simulink model "LoadLevel1_VF"  (R2023a)
settings: Solver=ode23tb  StartTime=0.0  StopTime=250  MaxStep=0.02  RelTol=1e-3  AbsTol=1e-5
undefined symbols (not defined in the file): a, Ac, Bc, Cc, D1, Dc, Delta, find_system, Fnom, gcbh, I21_init_imag, I21_init_real, Ibase1, Ibase2, Iw1A_init_mag, Iw1A_init_pha, Iw1B_init_mag, Iw1B_init_pha, Iw1C_init_mag, Iw1C_init_pha, Iw2A_init_mag, Iw2A_init_pha, Iw2B_init_mag, Iw2B_init_pha, Iw2C_init_mag, Iw2C_init_pha, j, kr, ks, Nmax, Pnom, psi, RegulatorDeadBand, RegulatorDelay, RegulatorVref, sps_rtmsupport, Vnom1, Vnom2, w, Z1pu, Z2pu, Ztpu
libraries: spsThreePhaseVIMeasurementLib x15, spsThreePhasePISectionLineLib x14, spsThreePhaseParallelRLCLoadLib x11, spsControlledCurrentSourceLib x6, spsThreePhaseTransformerTwoWindingsLib x5, spsThreePhaseBreakerLib x2, spsExcitationSystemLib x2, spsHydraulicTurbineandGovernorLib x2, spsSynchronousMachinepuStandardLib x2, spsThreePhaseSeriesRLCBranchLib x2, spsGroundLib x2, spsSequenceAnalyzerPhasorLib x1
(part 2 of 3)

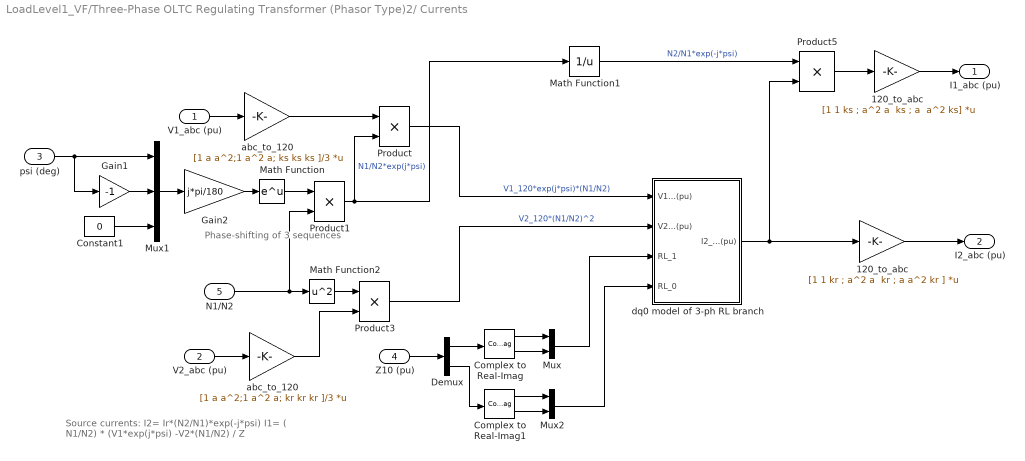
== system LoadLevel1_VF/Three-Phase OLTC Regulating Transformer (Phasor Type)2/ Currents  ==
  note: Phase-shifting
      | of 3 sequences
  note: Source currents:
      |
      | I2= Ir*(N2/N1)*exp(-j*psi)
      | I1= ( N1/N2) * (V1*exp(j*psi) -V2*(N1/N2) / Z
  V1_abc (pu) : Inport
  V2_abc (pu) : Inport  Port=2
  psi (deg) : Inport  Port=3
  Z10 (pu) : Inport  Port=4
  N1/N2 : Inport  Port=5
  120_to_abc : Gain  Gain="[1 1 kr ; a^2 a  kr ; a a^2 kr ]"  Multiplication=Matrix(K*u)  SaturateOnIntegerOverflow=on  OutDataTypeStr=Inherit: Same as input  ParamDataTypeStr=Inherit: Same as input
  "120_to_abc " : Gain  Gain="[1 1 ks ; a^2 a  ks ; a  a^2 ks]"  Multiplication=Matrix(K*u)  SaturateOnIntegerOverflow=on  OutDataTypeStr=Inherit: Same as input  ParamDataTypeStr=Inherit: Same as input
  Complex to Real-Imag : ComplexToRealImag
  Complex to Real-Imag1 : ComplexToRealImag
  Constant1 : Constant  Value=0
  Demux : Demux  Outputs=2
      settings: DisplayOption=none
  Gain1 : Gain  Gain=-1  SaturateOnIntegerOverflow=on  OutDataTypeStr=Inherit: Same as input  ParamDataTypeStr=Inherit: Same as input
  Gain2 : Gain  Gain=j*pi/180  SaturateOnIntegerOverflow=on  OutDataTypeStr=Inherit: Same as input  ParamDataTypeStr=Inherit: Same as input
  Math Function : Math  SignedPower=on
  Math Function1 : Math  Operator=reciprocal  SignedPower=on
  Math Function2 : Math  Operator=square  SignedPower=on
  Mux : Mux  Inputs=2
  Mux1 : Mux  Inputs=3
  Mux2 : Mux  Inputs=2
  Product : Product  SaturateOnIntegerOverflow=on  OutDataTypeStr=Inherit: Same as first input
  Product1 : Product  Inputs=**  SaturateOnIntegerOverflow=on  OutDataTypeStr=Inherit: Same as first input
  Product3 : Product  Inputs=**  SaturateOnIntegerOverflow=on  OutDataTypeStr=Inherit: Same as first input
  Product5 : Product  SaturateOnIntegerOverflow=on  OutDataTypeStr=Inherit: Same as first input
  abc_to_120 : Gain  Gain=[1 a a^2;1 a^2 a; ks ks ks ]/3  Multiplication=Matrix(K*u)  SaturateOnIntegerOverflow=on  OutDataTypeStr=Inherit: Same as input  ParamDataTypeStr=Inherit: Same as input
  "abc_to_120 " : Gain  Gain=[1 a a^2;1 a^2 a; kr kr kr ]/3  Multiplication=Matrix(K*u)  SaturateOnIntegerOverflow=on  OutDataTypeStr=Inherit: Same as input  ParamDataTypeStr=Inherit: Same as input
  dq0 model of 3-ph RL branch : Subsystem
  I1_abc (pu) : Outport  VectorParamsAs1DForOutWhenUnconnected=off
  "I2_abc (pu) " : Outport  Port=2  VectorParamsAs1DForOutWhenUnconnected=off
  wires:
  Gain2/1 -> Math Function/1
  Product/1 -> dq0 model of 3-ph RL branch/1(V1_120(pu))  "V1_120*exp(j*psi)*(N1/N2)"
  Product3/1 -> dq0 model of 3-ph RL branch/2(V2_120(pu))  "V2_120*(N1/N2)^2"
  N1/N2/1 -> Product1/2, Math Function2/1
  Product1/1 -> Math Function1/1, Product/2  "N1/N2*exp(j*psi)"
  Math Function/1 -> Product1/1
  V1_abc (pu)/1 -> abc_to_120/1
  V2_abc (pu)/1 -> "abc_to_120 "/1
  Product5/1 -> "120_to_abc "/1
  abc_to_120/1 -> Product/1
  Math Function1/1 -> Product5/1  "N2/N1*exp(-j*psi)"
  psi (deg)/1 -> Gain1/1, Mux1/1
  Mux1/1 -> Gain2/1
  Gain1/1 -> Mux1/2
  Constant1/1 -> Mux1/3
  "abc_to_120 "/1 -> Product3/2
  120_to_abc/1 -> "I2_abc (pu) "/1
  "120_to_abc "/1 -> I1_abc (pu)/1
  Z10 (pu)/1 -> Demux/1
  Demux/1 -> Complex to Real-Imag/1
  Demux/2 -> Complex to Real-Imag1/1
  Complex to Real-Imag/1 -> Mux/1
  Complex to Real-Imag/2 -> Mux/2
  Mux/1 -> dq0 model of 3-ph RL branch/3(RL_1)
  Complex to Real-Imag1/1 -> Mux2/1
  Complex to Real-Imag1/2 -> Mux2/2
  Mux2/1 -> dq0 model of 3-ph RL branch/4(RL_0)
  dq0 model of 3-ph RL branch/1(I2_120 (pu)) -> 120_to_abc/1, Product5/2
  Math Function2/1 -> Product3/1

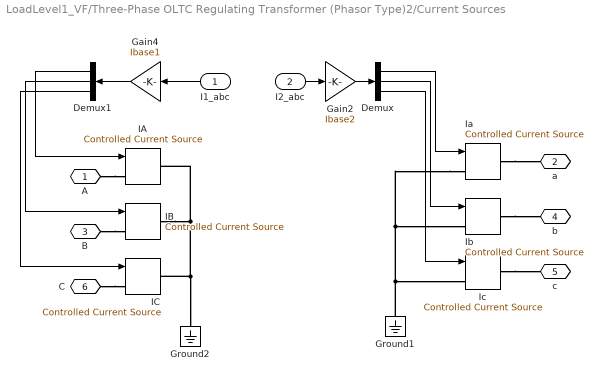
== system LoadLevel1_VF/Three-Phase OLTC Regulating Transformer (Phasor Type)2/Current Sources ==
  I1_abc : Inport
  I2_abc : Inport  Port=2
  Demux : Demux  Outputs=3
      settings: DisplayOption=none
  Demux1 : Demux  Outputs=3
      settings: DisplayOption=none
  Gain2 : Gain  Gain=Ibase2  SaturateOnIntegerOverflow=on  OutDataTypeStr=Inherit: Same as input  ParamDataTypeStr=Inherit: Same as input
  Gain4 : Gain  Gain=Ibase1  SaturateOnIntegerOverflow=on  OutDataTypeStr=Inherit: Same as input  ParamDataTypeStr=Inherit: Same as input
  Ground1 : spsGroundLib/Ground  LConnTagsString=a
  Ground2 : spsGroundLib/Ground  LConnTagsString=a
  IA : spsControlledCurrentSourceLib/Controlled Current Source  Initialize=on  Source_Type=AC  Amplitude=Iw1A_init_mag  Phase=Iw1A_init_pha  Frequency=Fnom  Measurements=None
  IB : spsControlledCurrentSourceLib/Controlled Current Source  Initialize=on  Source_Type=AC  Amplitude=Iw1B_init_mag  Phase=Iw1B_init_pha  Frequency=Fnom  Measurements=None
  IC : spsControlledCurrentSourceLib/Controlled Current Source  Initialize=on  Source_Type=AC  Amplitude=Iw1C_init_mag  Phase=Iw1C_init_pha  Frequency=Fnom  Measurements=None
  Ia : spsControlledCurrentSourceLib/Controlled Current Source  Initialize=on  Source_Type=AC  Amplitude=Iw2A_init_mag  Phase=Iw2A_init_pha  Frequency=Fnom  Measurements=None
  Ib : spsControlledCurrentSourceLib/Controlled Current Source  Initialize=on  Source_Type=AC  Amplitude=Iw2B_init_mag  Phase=Iw2B_init_pha  Frequency=Fnom  Measurements=None
  Ic : spsControlledCurrentSourceLib/Controlled Current Source  Initialize=on  Source_Type=AC  Amplitude=Iw2C_init_mag  Phase=Iw2C_init_pha  Frequency=Fnom  Measurements=None
  A : PMIOPort  Side=Left
  a : PMIOPort  Port=2  Side=Right
  B : PMIOPort  Port=3  Side=Left
  b : PMIOPort  Port=4  Side=Right
  c : PMIOPort  Port=5  Side=Right
  C : PMIOPort  Port=6  Side=Left
  wires:
  I1_abc/1 -> Gain4/1
  I2_abc/1 -> Gain2/1
  Demux/3 -> Ic/1
  Demux/2 -> Ib/1
  Demux/1 -> Ia/1
  Demux1/3 -> IC/1
  Demux1/2 -> IB/1
  Demux1/1 -> IA/1
  Gain2/1 -> Demux/1
  Gain4/1 -> Demux1/1
  connections:
  Ic/RConn1 -- c/RConn1
  Ib/RConn1 -- b/RConn1
  Ia/RConn1 -- a/RConn1
  C/RConn1 -- IC/LConn1
  B/RConn1 -- IB/LConn1
  A/RConn1 -- IA/LConn1
  Ia/LConn1 -- Ib/LConn1 -- Ic/LConn1 -- Ground1/LConn1
  IB/RConn1 -- IA/RConn1 -- IC/RConn1 -- Ground2/LConn1

== system LoadLevel1_VF/Three-Phase OLTC Regulating Transformer (Phasor Type)2/Tap Changer Control ==
  "Up " : Inport
  "Down " : Inport  Port=2
  Constant : Constant  Value=-1
  Constant1 : Constant
  Determine tap position : Subsystem
  Edge Detector : Subsystem  DialogController=POWERSYS.PowerSysDialog  mask(Edge Detector){model=Rising, ic=0}
      mask prompts: model "Edge:"; ic "Input at t = -eps:"
      mask help:
      | This block compares its present input to its previous input.
      |
      | If the input  is a logic signal (TRUE (1) or FALSE (0), the output is a one-step boolean signal TRUE  when  the specified edge (Rising, Falling or Either)  is detected.
      |
      | This block can also be used to detect the slope polarity of a continuous signal. For example, if the specified edge is  "Rising", the output is TRUE as long as the slope of the input signal is positive.
      |
      | The input value at time preceding t=0 is specified by the parameter "Input at t=-eps"
      mask init:
      | if model~=3,
      | 	x1 = (model -1)*20;
      |     x2 = (model -1)*60;
      | 	X1=[5,20,20,35]+25; Y1=[20+x2,20+x2,80-x2,80-x2];
      | 	X2=[5,20,35]+25;    Y2=[40+x1,60-x1,40+x1];
      | 	X3=[];X4=[];Y3=[];Y4=[];
      | else
      | 	x1 = 20;
      | 	x2 = 60;
      | 	X1=[5,20,20,35]+8; Y1=[20,20,80,80];
      | 	X2=[5,20,35]+8;    Y2=[40,60,40];
      | 	X3=[5,20,20,35]+53; Y3=[20+x2,20+x2,80-x2,80-x2];
      | 	X4=[5,20,35]+53;    Y4=[40+x1,60-x1,40+x1];
      | end
      | power_initmask();
      mask Help: This block is part of a subset of blocks in the Extras library that does not have documentation associated with it, other than the block mask description.
      mask TypeOptions model: Rising | Falling | Either
      mask Display: plot(0,0,100,100, X1,Y1,X2,Y2,X3,Y3,X4,Y4);
  Logical Operator : Logic  Operator=OR  AllPortsSameDT=off
  Logical Operator1 : Logic  AllPortsSameDT=off
  Mechanical Delay : TransportDelay  DelayTime=MecDelay  InitialOutput=InitialPosition
  Memory : Memory  InitialCondition=1  InheritSampleTime=on
  Relational Operator : RelationalOperator  Operator===  OutDataTypeStr=float('double')  InputSameDT=off
  Switch : Switch  Threshold=0.5  InputSameDT=off
  TapNo : Outport  VectorParamsAs1DForOutWhenUnconnected=off
  Ready : Outport  Port=2  VectorParamsAs1DForOutWhenUnconnected=off
  wires:
  Edge Detector/1(Out) -> Logical Operator1/2
  Logical Operator/1 -> Edge Detector/1(In)
  Memory/1 -> Ready/1, Logical Operator1/1
  Relational Operator/1 -> Memory/1
  Determine tap position/1(TapNo) -> Relational Operator/1, Mechanical Delay/1
  Switch/1 -> Determine tap position/1(NewTap)
  Constant1/1 -> Switch/3
  Constant/1 -> Switch/1
  "Down "/1 -> Switch/2, Logical Operator/2
  "Up "/1 -> Logical Operator/1
  Logical Operator1/1 -> Determine tap position/Trigger
  Mechanical Delay/1 -> Relational Operator/2, TapNo/1

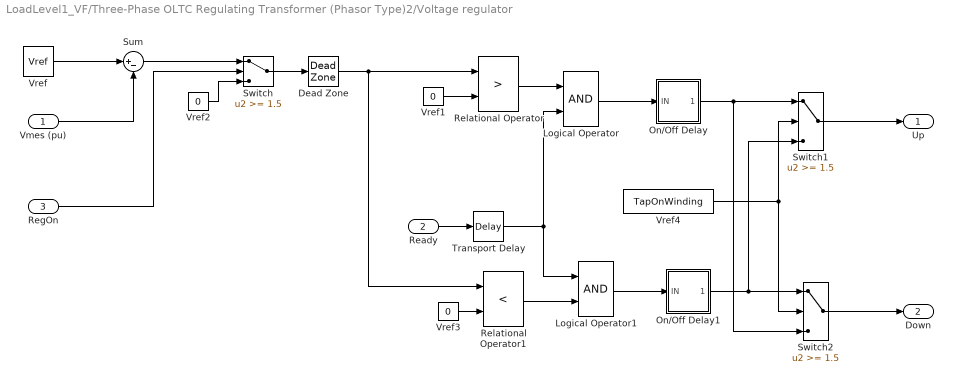
== system LoadLevel1_VF/Three-Phase OLTC Regulating Transformer (Phasor Type)2/Voltage regulator ==
  Vmes (pu) : Inport
  Ready : Inport  Port=2
  RegOn : Inport  Port=3
  Dead Zone : DeadZone  LowerValue=-DeadBand/2  UpperValue=+DeadBand/2
  Logical Operator : Logic  AllPortsSameDT=off
  Logical Operator1 : Logic  AllPortsSameDT=off
  On/Off Delay : Subsystem  DialogController=POWERSYS.PowerSysDialog  mask(On/Off Delay){type_delay=On delay, delay=TimeDelay, ic=0}
      mask prompts: type_delay "Type:"; delay "Time delay:"; ic "Input at t = -eps (0/1):"
      mask help:
      | Apply a delay on the input signal when the input changes to TRUE (1) or FALSE (0).
      |
      | On delay: When the input becomes TRUE, the output becomes TRUE after the specified time delay as long as the input is still TRUE. If the input becomes FALSE before the time delay has expired , the output stays FALSE.
      |
      | Off delay: When the input becomes FALSE, the output becomes FALSE after the specified time delay as long as the input is still FALSE. If the input becomes TRUE before the time delay has expired , the output stays TRUE.
      |
      | The input value (0/1) at time preceding t=0 is specified by the parameter "input at t = -eps".
      mask init:
      | str=sprintf('%g %c',delay,'s');
      | power_initmask();
      mask Help: This block is part of a subset of blocks in the Extras library that does not have documentation associated with it, other than the block mask description.
      mask TypeOptions type_delay: On delay | Off delay
      mask Display:
      | plot(0,0,100,100,[10,10,10,90,90,90],[60,40,50,50,40,60]);
      | text(25+(type_delay-1)*50,80,'t');
      | text(15,20,str);
  On/Off Delay1 : Subsystem  DialogController=POWERSYS.PowerSysDialog  mask(On/Off Delay){type_delay=On delay, delay=TimeDelay, ic=0}
      mask prompts: type_delay "Type:"; delay "Time delay:"; ic "Input at t = -eps (0/1):"
      mask help:
      | Apply a delay on the input signal when the input changes to TRUE (1) or FALSE (0).
      |
      | On delay: When the input becomes TRUE, the output becomes TRUE after the specified time delay as long as the input is still TRUE. If the input becomes FALSE before the time delay has expired , the output stays FALSE.
      |
      | Off delay: When the input becomes FALSE, the output becomes FALSE after the specified time delay as long as the input is still FALSE. If the input becomes TRUE before the time delay has expired , the output stays TRUE.
      |
      | The input value (0/1) at time preceding t=0 is specified by the parameter "input at t = -eps".
      mask init:
      | str=sprintf('%g %c',delay,'s');
      | power_initmask();
      mask Help: This block is part of a subset of blocks in the Extras library that does not have documentation associated with it, other than the block mask description.
      mask TypeOptions type_delay: On delay | Off delay
      mask Display:
      | plot(0,0,100,100,[10,10,10,90,90,90],[60,40,50,50,40,60]);
      | text(25+(type_delay-1)*50,80,'t');
      | text(15,20,str);
  Relational Operator : RelationalOperator  Operator=>  InputSameDT=off
  Relational Operator1 : RelationalOperator  Operator=<  InputSameDT=off
  Sum : Sum  Inputs=|+-  SaturateOnIntegerOverflow=on
  Switch : Switch  Threshold=1.5  InputSameDT=off
  Switch1 : Switch  Threshold=1.5  InputSameDT=off
  Switch2 : Switch  Threshold=1.5  InputSameDT=off
  Transport Delay : TransportDelay  DelayTime=3/60  InitialOutput=1
  Vref : Constant  Value=Vref
  Vref1 : Constant  Value=0
  Vref2 : Constant  Value=0
  Vref3 : Constant  Value=0
  Vref4 : Constant  Value=TapOnWinding
  "Up " : Outport  VectorParamsAs1DForOutWhenUnconnected=off
  "Down " : Outport  Port=2  VectorParamsAs1DForOutWhenUnconnected=off
  wires:
  Vref4/1 -> Switch2/2, Switch1/2
  Switch2/1 -> "Down "/1
  On/Off Delay1/1(OUT) -> Switch1/3, Switch2/1
  Switch1/1 -> "Up "/1
  On/Off Delay/1(OUT) -> Switch2/3, Switch1/1
  Vref2/1 -> Switch/3
  RegOn/1 -> Switch/2
  Switch/1 -> Dead Zone/1
  Sum/1 -> Switch/1
  Vref/1 -> Sum/1
  Vmes (pu)/1 -> Sum/2
  Dead Zone/1 -> Relational Operator1/1, Relational Operator/1
  Vref1/1 -> Relational Operator/2
  Relational Operator/1 -> Logical Operator/1
  Ready/1 -> Transport Delay/1
  Logical Operator/1 -> On/Off Delay/1(IN)
  Transport Delay/1 -> Logical Operator/2, Logical Operator1/1
  Vref3/1 -> Relational Operator1/2
  Relational Operator1/1 -> Logical Operator1/2
  Logical Operator1/1 -> On/Off Delay1/1(IN)

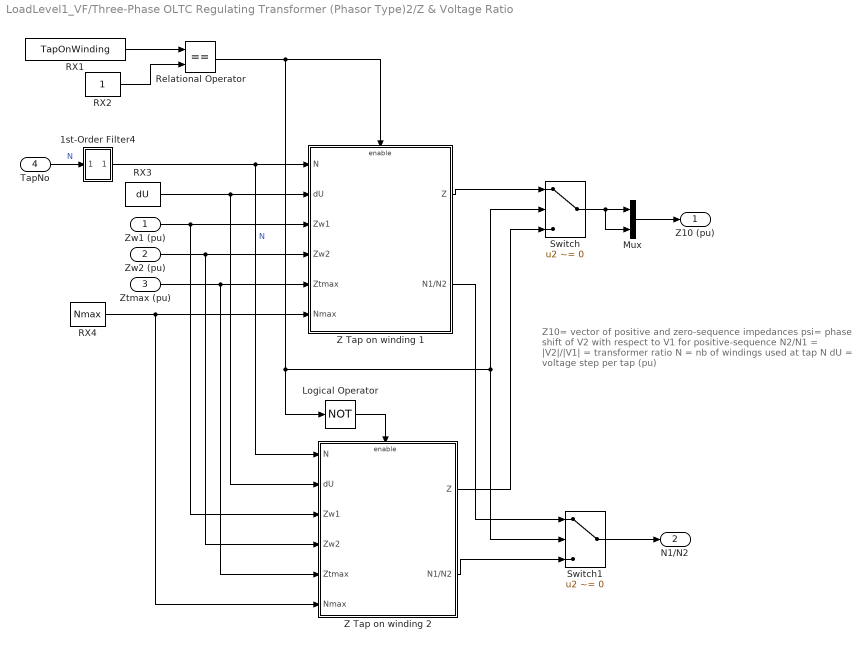
== system LoadLevel1_VF/Three-Phase OLTC Regulating Transformer (Phasor Type)2/Z & Voltage Ratio ==
  note: Z10= vector of positive and zero-sequence impedances
      | psi= phase shift of  V2 with respect to V1 for positive-sequence
      | N2/N1 =  |V2|/|V1| = transformer ratio
      | N = nb of windings used at tap N
      | dU = voltage step  per tap (pu)
  Zw1 (pu) : Inport
  Zw2 (pu) : Inport  Port=2
  Ztmax (pu) : Inport  Port=3
  TapNo : Inport  Port=4
  1st-Order Filter4 : Subsystem  DialogController=POWERSYS.PowerSysDialog  mask(First-Order Filter){FilterType=Lowpass, Tc=1/Fnom, Initialize=on, Vac_Init=[0 0  Fnom], Vdc_Init=InitialTap, PlotResponse=off, param1=[1 500 1]}
      mask prompts: FilterType "Filter Type:"; Tc "Time constant (s):"; Initialize "Initialize filter states"; Vac_Init "AC initial input: [ Mag  Phase(degrees)  Freq(Hz) ]"; Vdc_Init "DC Initial input:"; PlotResponse "Plot filter response"; param1 "Frequency range(Hz) : [Start  End  Inc.]"
      mask init:
      | switch FilterType
      | case 1, % Lowpass
      |        X=[0 1 2 3 4];
      |        Y=[-2 -2 -3 -4 -4];
      |        numc=1;
      |        denc=[Tc 1];
      |  case 2,   % Highpass
      |        X=[0 1 2 3 4];
      |        Y=[-4 -4 -3 -2 -2];
      |         numc=[1 0];
      |         denc=[1 1/Tc];
      | end
      | %
      | [Ac,Bc,Cc,Dc]=tf2ss(numc,denc);
      | %
      | %
      | if Initialize==1  % Compute initial conditions on states
      | u1=Vac_Init(1)*exp(j*Vac_Init(2)*pi/180);
      | u2=Vdc_Init*exp(j*90*pi/180);
      | u=u1+u2;
      | u0=imag(u); % input at  t=0;
      | I=eye(size(Ac));
      | sI1=I*j*(2*pi*Vac_Init(3));
      | sI2=I*j*0;
      | x=inv(sI1-Ac)*Bc*u1 + inv(sI2-Ac)*Bc*u2;
      | x0c=imag(x);
      | else
      | x0c=0;
      | end
      | %
      | if PlotResponse==1 % Plot frequency and step response
      | t=[0:Tc/1000:7*Tc];
      | f=param1(1):param1(3):param1(2);
      | w=2*pi*f;
      | switch FilterType
      | 	case 1, % Lowpass
      | 		Ystep=1 - exp(-t/Tc);
      | 		RepFreq=1./(1+Tc*j.*w);
      | 	case 2,   % Highpass
      | 		Ystep=exp(-t/Tc);
      | 		RepFreq=1./(1 + (1./(Tc*j.*w)));
      | end
      | %
      | Mag=abs(RepFreq);
      | Pha=angle(RepFreq)*180/pi;
      | %
      | figure(1)
      | subplot(2,1,1)
      | plot(f,Mag)
      | grid
      | title('Bode Diagram')
      | ylabel('Magnitude')
      | subplot(2,1,2)
      | plot(f,Pha)
      | ylabel('Phase (deg)')
      | xlabel('Frequency (Hz)')
      | grid
      | figure(2)
      | plot(t,Ystep)
      | grid
      | ylabel('Amplitude')
      | xlabel('Time (s)')
      | title('Step Response')
      | end
      | power_initmask();
      mask Help: This block is part of a subset of blocks in the Extras library that does not have documentation associated with it, other than the block mask description.
      mask TypeOptions FilterType: Lowpass | Highpass
      mask Callback Initialize: %parametres=get_param(gcb,'MaskValues');p3=parametres{3};p6=parametres{6};if strcmp(p3,'on');param4='on';param5='on';else;param4='off';param5='off';end;if strcmp(p6,'on');param7='on';else;param7='off';end;visible={'on','on','on',param4,param5,'on',param7};set_param(gcb,'MaskVisibilities',visible)
      mask Callback PlotResponse: %parametres=get_param(gcb,'MaskValues');p3=parametres{3};p6=parametres{6};if strcmp(p3,'on');param4='on';param5='on';else;param4='off';param5='off';end;if strcmp(p6,'on');param7='on';else;param7='off';end;visible={'on','on','on',param4,param5,'on',param7};set_param(gcb,'MaskVisibilities',visible)
      mask Display: plot(X,Y);
  Logical Operator : Logic  Operator=NOT  AllPortsSameDT=off
  Mux : Mux  Inputs=2
  RX1 : Constant  Value=TapOnWinding
  RX2 : Constant
  RX3 : Constant  Value=dU
  RX4 : Constant  Value=Nmax
  Relational Operator : RelationalOperator  Operator===  InputSameDT=off
  Switch : Switch  Criteria=u2 ~= 0  Threshold=0.5  InputSameDT=off
  Switch1 : Switch  Criteria=u2 ~= 0  Threshold=0.5  InputSameDT=off
  Z Tap on winding 1 : Subsystem
  Z Tap on winding 2 : Subsystem
  "Z10 (pu) " : Outport  VectorParamsAs1DForOutWhenUnconnected=off
  N1/N2 : Outport  Port=2  VectorParamsAs1DForOutWhenUnconnected=off
  wires:
  RX4/1 -> Z Tap on winding 2/6(Nmax), Z Tap on winding 1/6(Nmax)
  TapNo/1 -> 1st-Order Filter4/1(In)  "N"
  1st-Order Filter4/1(Out) -> Z Tap on winding 1/1(N), Z Tap on winding 2/1(N)  "N"
  Zw2 (pu)/1 -> Z Tap on winding 1/4(Zw2), Z Tap on winding 2/4(Zw2)
  Zw1 (pu)/1 -> Z Tap on winding 1/3(Zw1), Z Tap on winding 2/3(Zw1)
  RX1/1 -> Relational Operator/1
  RX2/1 -> Relational Operator/2
  Relational Operator/1 -> Z Tap on winding 1/Enable, Logical Operator/1, Switch/2, Switch1/2
  Logical Operator/1 -> Z Tap on winding 2/Enable
  Z Tap on winding 1/1(Z) -> Switch/1
  Z Tap on winding 2/1(Z) -> Switch/3
  Z Tap on winding 1/2(N1/N2) -> Switch1/1
  Z Tap on winding 2/2(N1/N2) -> Switch1/3
  Switch1/1 -> N1/N2/1
  Ztmax (pu)/1 -> Z Tap on winding 1/5(Ztmax), Z Tap on winding 2/5(Ztmax)
  RX3/1 -> Z Tap on winding 1/2(dU), Z Tap on winding 2/2(dU)
  Switch/1 -> Mux/1, Mux/2
  Mux/1 -> "Z10 (pu) "/1

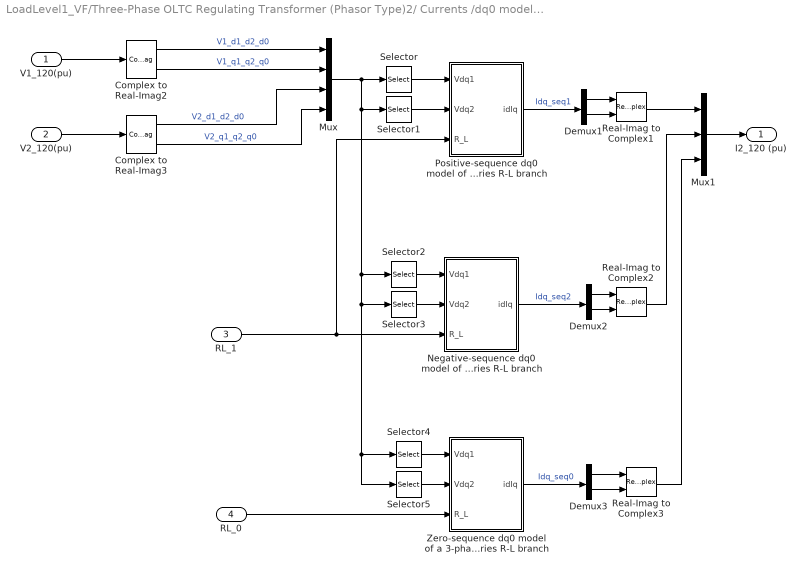
== system LoadLevel1_VF/Three-Phase OLTC Regulating Transformer (Phasor Type)2/ Currents /dq0 model of 3-ph RL branch ==
  V1_120(pu) : Inport
  V2_120(pu) : Inport  Port=2
  RL_1 : Inport  Port=3
  RL_0 : Inport  Port=4
  Complex to Real-Imag2 : ComplexToRealImag
  Complex to Real-Imag3 : ComplexToRealImag
  Demux1 : Demux  Outputs=2
      settings: DisplayOption=none
  Demux2 : Demux  Outputs=2
      settings: DisplayOption=none
  Demux3 : Demux  Outputs=2
      settings: DisplayOption=none
  Mux : Mux
  Mux1 : Mux  Inputs=3
  Negative-sequence dq0 model of a 3-phase series R-L branch : Subsystem
  Positive-sequence dq0 model of a 3-phase series R-L branch : Subsystem
  Real-Imag to Complex1 : RealImagToComplex
  Real-Imag to Complex2 : RealImagToComplex
  Real-Imag to Complex3 : RealImagToComplex
  Selector : Selector  InputPortWidth=12  IndexOptions=Index vector (dialog)  Indices=[1 4]  OutputSizes=1
  Selector1 : Selector  InputPortWidth=12  IndexOptions=Index vector (dialog)  Indices=[7 10]  OutputSizes=1
  Selector2 : Selector  InputPortWidth=12  IndexOptions=Index vector (dialog)  Indices=[1 4]+1  OutputSizes=1
  Selector3 : Selector  InputPortWidth=12  IndexOptions=Index vector (dialog)  Indices=[7 10]+1  OutputSizes=1
  Selector4 : Selector  InputPortWidth=12  IndexOptions=Index vector (dialog)  Indices=[1 4]+2  OutputSizes=1
  Selector5 : Selector  InputPortWidth=12  IndexOptions=Index vector (dialog)  Indices=[7 10]+2  OutputSizes=1
  Zero-sequence dq0 model of a 3-phase series R-L branch : Subsystem
  I2_120 (pu) : Outport  VectorParamsAs1DForOutWhenUnconnected=off
  wires:
  Positive-sequence dq0 model of a 3-phase series R-L branch/1(idIq) -> Demux1/1  "Idq_seq1"
  V1_120(pu)/1 -> Complex to Real-Imag2/1
  V2_120(pu)/1 -> Complex to Real-Imag3/1
  Selector/1 -> Positive-sequence dq0 model of a 3-phase series R-L branch/1(Vdq1)
  Selector1/1 -> Positive-sequence dq0 model of a 3-phase series R-L branch/2(Vdq2)
  Mux/1 -> Selector/1, Selector1/1, Selector2/1, Selector3/1, Selector4/1, Selector5/1
  Selector2/1 -> Negative-sequence dq0 model of a 3-phase series R-L branch/1(Vdq1)
  Selector3/1 -> Negative-sequence dq0 model of a 3-phase series R-L branch/2(Vdq2)
  Selector4/1 -> Zero-sequence dq0 model of a 3-phase series R-L branch/1(Vdq1)
  Negative-sequence dq0 model of a 3-phase series R-L branch/1(idIq) -> Demux2/1  "Idq_seq2"
  Zero-sequence dq0 model of a 3-phase series R-L branch/1(idIq) -> Demux3/1  "Idq_seq0"
  Complex to Real-Imag2/1 -> Mux/1  "V1_d1_d2_d0"
  Complex to Real-Imag2/2 -> Mux/2  "V1_q1_q2_q0"
  Complex to Real-Imag3/1 -> Mux/3  "V2_d1_d2_d0"
  Complex to Real-Imag3/2 -> Mux/4  "V2_q1_q2_q0"
  RL_1/1 -> Positive-sequence dq0 model of a 3-phase series R-L branch/3(R_L), Negative-sequence dq0 model of a 3-phase series R-L branch/3(R_L)
  Selector5/1 -> Zero-sequence dq0 model of a 3-phase series R-L branch/2(Vdq2)
  RL_0/1 -> Zero-sequence dq0 model of a 3-phase series R-L branch/3(R_L)
  Demux1/2 -> Real-Imag to Complex1/2
  Demux1/1 -> Real-Imag to Complex1/1
  Real-Imag to Complex1/1 -> Mux1/1
  Demux2/2 -> Real-Imag to Complex2/2
  Demux2/1 -> Real-Imag to Complex2/1
  Real-Imag to Complex2/1 -> Mux1/2
  Demux3/2 -> Real-Imag to Complex3/2
  Demux3/1 -> Real-Imag to Complex3/1
  Real-Imag to Complex3/1 -> Mux1/3
  Mux1/1 -> I2_120 (pu)/1

== system LoadLevel1_VF/Three-Phase OLTC Regulating Transformer (Phasor Type)2/Tap Changer Control/Determine tap position ==
  NewTap : Inport
  Trigger : TriggerPort  VariantControl=Variant
  Memory : Memory  InitialCondition=InitialPosition  InheritSampleTime=on
  Saturation : Saturate  UpperLimit=MinMaxTap(2)  LowerLimit=MinMaxTap(1)
  Sum : Sum  Inputs=|++  SaturateOnIntegerOverflow=on
  TapNo : Outport  InitialOutput=InitialPosition  VectorParamsAs1DForOutWhenUnconnected=off
  wires:
  Saturation/1 -> Memory/1, TapNo/1
  Memory/1 -> Sum/2
  Sum/1 -> Saturation/1
  NewTap/1 -> Sum/1

== system LoadLevel1_VF/Three-Phase OLTC Regulating Transformer (Phasor Type)2/Tap Changer Control/Edge Detector ==
  note: Edge or Slope Detector
  In : Inport
  Constant1 : Constant  Value=model
  Demux : Demux  Outputs=2
      settings: DisplayOption=none
  Logical Operator1 : Logic  Operator=OR
  Memory : Memory  InitialCondition=ic  LinearizeAsDelay=on
  Multiport Switch : MultiPortSwitch  InputSameDT=off
  NEGATIVE Edge : Subsystem  TreatAsAtomicUnit=on
  POSITIVE Edge : Subsystem  TreatAsAtomicUnit=on
  either edge : Constant  Value=[1 1]
  neg. edge : Constant  Value=[0 1]
  pos. edge : Constant  Value=[1 0]
  Out : Outport  VectorParamsAs1DForOutWhenUnconnected=off
  wires:
  Logical Operator1/1 -> Out/1
  NEGATIVE Edge/1(OUT) -> Logical Operator1/2
  POSITIVE Edge/1(OUT) -> Logical Operator1/1
  Memory/1 -> POSITIVE Edge/2(IN previous), NEGATIVE Edge/2(IN previous)
  In/1 -> POSITIVE Edge/1(IN), NEGATIVE Edge/1(IN), Memory/1
  pos. edge/1 -> Multiport Switch/2
  neg. edge/1 -> Multiport Switch/3
  Constant1/1 -> Multiport Switch/1
  Multiport Switch/1 -> Demux/1
  Demux/1 -> POSITIVE Edge/Enable
  Demux/2 -> NEGATIVE Edge/Enable
  either edge/1 -> Multiport Switch/4

== system LoadLevel1_VF/Three-Phase OLTC Regulating Transformer (Phasor Type)2/Voltage regulator/On//Off Delay ==
  note: Silvano Casoria
      | Power System Simulation Laboratory
      | IREQ, Hydro-Quebc
  note: On/Off Delay
  IN : Inport
  Clock : Clock
  Constant : Constant
  Constant1 : Constant  Value=delay
  Constant2 : Constant  Value=type_delay
  Data Type Conversion1 : DataTypeConversion  OutDataTypeStr=boolean
  Logical Operator1 : Logic  Operator=OR
  Logical Operator2 : Logic  Operator=NOT  Inputs=1
  OFF Delay : Subsystem  TreatAsAtomicUnit=on
  ON Delay : Subsystem  TreatAsAtomicUnit=on
  Relational Operator1 : RelationalOperator  Operator===
  OUT : Outport  VectorParamsAs1DForOutWhenUnconnected=off
  wires:
  Data Type Conversion1/1 -> OFF Delay/1(IN), ON Delay/1(IN)
  Constant/1 -> Relational Operator1/2
  Relational Operator1/1 -> ON Delay/Enable, Logical Operator2/1
  Constant2/1 -> Relational Operator1/1
  Logical Operator2/1 -> OFF Delay/Enable
  OFF Delay/1(OUT) -> Logical Operator1/2
  ON Delay/1(OUT) -> Logical Operator1/1
  Logical Operator1/1 -> OUT/1
  Constant1/1 -> ON Delay/3(DELAY), OFF Delay/3(DELAY)
  IN/1 -> Data Type Conversion1/1
  Clock/1 -> OFF Delay/2(clock), ON Delay/2(clock)

== system LoadLevel1_VF/Three-Phase OLTC Regulating Transformer (Phasor Type)2/Voltage regulator/On//Off Delay1 ==
  note: Silvano Casoria
      | Power System Simulation Laboratory
      | IREQ, Hydro-Quebc
  note: On/Off Delay
  IN : Inport
  Clock : Clock
  Constant : Constant
  Constant1 : Constant  Value=delay
  Constant2 : Constant  Value=type_delay
  Data Type Conversion1 : DataTypeConversion  OutDataTypeStr=boolean
  Logical Operator1 : Logic  Operator=OR
  Logical Operator2 : Logic  Operator=NOT  Inputs=1
  OFF Delay : Subsystem  TreatAsAtomicUnit=on
  ON Delay : Subsystem  TreatAsAtomicUnit=on
  Relational Operator1 : RelationalOperator  Operator===
  OUT : Outport  VectorParamsAs1DForOutWhenUnconnected=off
  wires:
  Data Type Conversion1/1 -> OFF Delay/1(IN), ON Delay/1(IN)
  Constant/1 -> Relational Operator1/2
  Relational Operator1/1 -> ON Delay/Enable, Logical Operator2/1
  Constant2/1 -> Relational Operator1/1
  Logical Operator2/1 -> OFF Delay/Enable
  OFF Delay/1(OUT) -> Logical Operator1/2
  ON Delay/1(OUT) -> Logical Operator1/1
  Logical Operator1/1 -> OUT/1
  Constant1/1 -> ON Delay/3(DELAY), OFF Delay/3(DELAY)
  IN/1 -> Data Type Conversion1/1
  Clock/1 -> OFF Delay/2(clock), ON Delay/2(clock)

== system LoadLevel1_VF/Three-Phase OLTC Regulating Transformer (Phasor Type)2/Z & Voltage Ratio/1st-Order Filter4 ==
  In : Inport
  State-Space : StateSpace  A=Ac  B=Bc  C=Cc  D=Dc  InitialCondition=x0c
  Out : Outport  InitialOutput=0  VectorParamsAs1DForOutWhenUnconnected=off
  wires:
  In/1 -> State-Space/1
  State-Space/1 -> Out/1

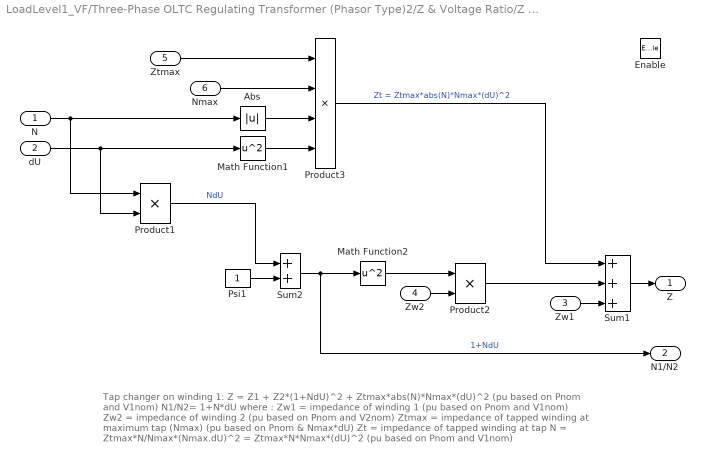
== system LoadLevel1_VF/Three-Phase OLTC Regulating Transformer (Phasor Type)2/Z & Voltage Ratio/Z Tap on winding 1 ==
  note: Tap changer on winding 1:
      | Z = Z1  + Z2*(1+NdU)^2 +  Ztmax*abs(N)*Nmax*(dU)^2       (pu based on Pnom and V1nom)
      | N1/N2= 1+N*dU
      |
      | where :
      | Zw1   =  impedance of winding 1 (pu based on Pnom and V1nom)
      | Zw2   =  impedance of winding 2 (pu based on Pnom and V2nom)
      | Ztmax =   impedance of tapped winding at maximum tap (Nmax)     (pu  based on  Pnom & Nmax*dU)
      | Zt =  impedance of tapped winding at tap N
      |      = Ztmax*N/Nmax*(Nmax.dU)^2 = Ztmax*N*Nmax*(dU)^2              (pu based on Pnom and V1nom)
  N : Inport
  dU : Inport  Port=2
  Zw1 : Inport  Port=3
  Zw2 : Inport  Port=4
  Ztmax : Inport  Port=5
  Nmax : Inport  Port=6
  Enable : EnablePort  PropagateVarSize=During execution
  Abs : Abs  SaturateOnIntegerOverflow=off
  Math Function1 : Math  Operator=square  SignedPower=on
  Math Function2 : Math  Operator=square  SignedPower=on
  Product1 : Product  SaturateOnIntegerOverflow=on  OutDataTypeStr=Inherit: Same as first input
  Product2 : Product  SaturateOnIntegerOverflow=on  OutDataTypeStr=Inherit: Same as first input
  Product3 : Product  Inputs=****  SaturateOnIntegerOverflow=on  OutDataTypeStr=Inherit: Same as first input
  Psi1 : Constant
  Sum1 : Sum  Inputs=+++  SaturateOnIntegerOverflow=on
  Sum2 : Sum  SaturateOnIntegerOverflow=on
  Z : Outport  VectorParamsAs1DForOutWhenUnconnected=off
  N1/N2 : Outport  Port=2  VectorParamsAs1DForOutWhenUnconnected=off
  wires:
  Nmax/1 -> Product3/2
  Math Function1/1 -> Product3/4
  Ztmax/1 -> Product3/1
  Product2/1 -> Sum1/2
  Math Function2/1 -> Product2/1
  Sum1/1 -> Z/1
  Zw2/1 -> Product2/2
  Zw1/1 -> Sum1/3
  Psi1/1 -> Sum2/2
  Sum2/1 -> Math Function2/1, N1/N2/1  "1+NdU"
  N/1 -> Product1/1, Abs/1
  dU/1 -> Product1/2, Math Function1/1
  Product1/1 -> Sum2/1  "NdU"
  Product3/1 -> Sum1/1  "Zt = Ztmax*abs(N)*Nmax*(dU)^2"
  Abs/1 -> Product3/3

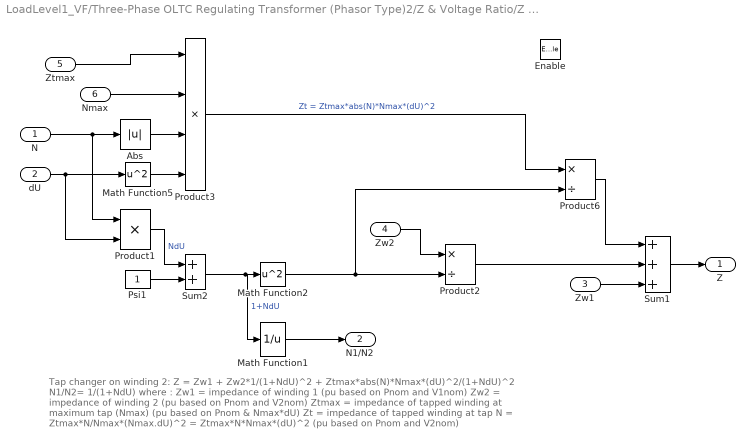
== system LoadLevel1_VF/Three-Phase OLTC Regulating Transformer (Phasor Type)2/Z & Voltage Ratio/Z Tap on winding 2 ==
  note: Tap changer on winding 2:
      | Z = Zw1  + Zw2*1/(1+NdU)^2 +  Ztmax*abs(N)*Nmax*(dU)^2/(1+NdU)^2
      | N1/N2= 1/(1+NdU)
      |
      | where :
      | Zw1   =  impedance of winding 1 (pu based on Pnom and V1nom)
      | Zw2   =  impedance of winding 2 (pu based on Pnom and V2nom)
      | Ztmax = impedance of tapped winding at maximum tap (Nmax)     (pu  based on  Pnom & Nmax*dU)
      | Zt =  impedance of tapped winding at tap N
      |      = Ztmax*N/Nmax*(Nmax.dU)^2 = Ztmax*N*Nmax*(dU)^2             (pu based on Pnom and V2nom)
  N : Inport
  dU : Inport  Port=2
  Zw1 : Inport  Port=3
  Zw2 : Inport  Port=4
  Ztmax : Inport  Port=5
  Nmax : Inport  Port=6
  Enable : EnablePort  PropagateVarSize=During execution
  Abs : Abs  SaturateOnIntegerOverflow=off
  Math Function1 : Math  Operator=reciprocal  SignedPower=on
  Math Function2 : Math  Operator=square  SignedPower=on
  Math Function5 : Math  Operator=square  SignedPower=on
  Product1 : Product  SaturateOnIntegerOverflow=on  OutDataTypeStr=Inherit: Same as first input
  Product2 : Product  Inputs=*/  SaturateOnIntegerOverflow=on  OutDataTypeStr=Inherit: Same as first input
  Product3 : Product  Inputs=****  SaturateOnIntegerOverflow=on  OutDataTypeStr=Inherit: Same as first input
  Product6 : Product  Inputs=*/  SaturateOnIntegerOverflow=on  OutDataTypeStr=Inherit: Same as first input
  Psi1 : Constant
  Sum1 : Sum  Inputs=+++  SaturateOnIntegerOverflow=on
  Sum2 : Sum  SaturateOnIntegerOverflow=on
  Z : Outport  VectorParamsAs1DForOutWhenUnconnected=off
  N1/N2 : Outport  Port=2  VectorParamsAs1DForOutWhenUnconnected=off
  wires:
  Math Function5/1 -> Product3/4
  Nmax/1 -> Product3/2
  Ztmax/1 -> Product3/1
  Product1/1 -> Sum2/1  "NdU"
  dU/1 -> Product1/2, Math Function5/1
  N/1 -> Product1/1, Abs/1
  Sum2/1 -> Math Function2/1, Math Function1/1  "1+NdU"
  Psi1/1 -> Sum2/2
  Zw1/1 -> Sum1/3
  Sum1/1 -> Z/1
  Product2/1 -> Sum1/2
  Zw2/1 -> Product2/1
  Math Function2/1 -> Product2/2, Product6/2
  Product3/1 -> Product6/1  "Zt = Ztmax*abs(N)*Nmax*(dU)^2"
  Product6/1 -> Sum1/1
  Math Function1/1 -> N1/N2/1
  Abs/1 -> Product3/3

== system LoadLevel1_VF/Three-Phase OLTC Regulating Transformer (Phasor Type)2/ Currents /dq0 model of 3-ph RL branch/Negative-sequence dq0 model of a 3-phase series R-L branch ==
  note: where w = 2*pi*Fnom (Hz)
  note: Vq1 - Vq2 = [ R * Iq ] + [ L* w * Id ] + [ L * d/dt (Iq) ]
  note: ==========================================================================================
  note: I --->
  note: V2
  note: V1
  note: o--------| R |---| L |-------o
  note: Vd1 - Vd2 = [ R * Id ] - [ L* w * Iq ] + [ L * d/dt (Id) ]
  note: where w = 2*pi*Fnom (Hz)
  note: Iq = [ w / ( L * s ) ] * [ Vq1 - Vq2 - ( R * Iq ) - ( L * Id ) ]
  note: Id = [ w / ( L * s ) ] * [ Vd1 - Vd2 - ( R * Id ) + ( L * Iq ) ]
  note: d-q axis model of a 3-phase series R-L branch
  note: Using Laplace transform and per unit (pu) quantities :
  Vdq1 : Inport
  Vdq2 : Inport  Port=2
  R_L : Inport  Port=3
  Demux3 : Demux  Outputs=2
      settings: DisplayOption=none
  Integrator : Integrator
  Product : Product  SaturateOnIntegerOverflow=on  OutDataTypeStr=Inherit: Same as first input
  Product1 : Product  SaturateOnIntegerOverflow=on  OutDataTypeStr=Inherit: Same as first input
  Product2 : Product  Inputs=*/  SaturateOnIntegerOverflow=on  OutDataTypeStr=Inherit: Same as first input
  R_choke2 : Gain  Gain=[1 -1]  SaturateOnIntegerOverflow=on  OutDataTypeStr=Inherit: Same as input  ParamDataTypeStr=Inherit: Same as input
  R_choke3 : Gain  Gain=w  SaturateOnIntegerOverflow=on  OutDataTypeStr=Inherit: Same as input  ParamDataTypeStr=Inherit: Same as input
  Selector : Selector  InputPortWidth=2  IndexOptions=Index vector (dialog)  Indices=[2 1]  OutputSizes=1
  Sum : Sum  Inputs=+--+  SaturateOnIntegerOverflow=on
  idIq : Outport  VectorParamsAs1DForOutWhenUnconnected=off
  wires:
  Demux3/1 -> Product/2
  Demux3/2 -> Product1/2, Product2/2
  R_L/1 -> Demux3/1
  Product2/1 -> Integrator/1
  R_choke3/1 -> Product2/1
  Selector/1 -> Product1/1
  Integrator/1 -> Product/1, Selector/1, idIq/1
  Sum/1 -> R_choke3/1
  Product1/1 -> R_choke2/1
  R_choke2/1 -> Sum/4
  Product/1 -> Sum/3
  Vdq2/1 -> Sum/2
  Vdq1/1 -> Sum/1

== system LoadLevel1_VF/Three-Phase OLTC Regulating Transformer (Phasor Type)2/ Currents /dq0 model of 3-ph RL branch/Positive-sequence dq0 model of a 3-phase series R-L branch ==
  note: Using Laplace transform and per unit (pu) quantities :
  note: d-q axis model of a 3-phase series R-L branch
  note: Id = [ w / ( L * s ) ] * [ Vd1 - Vd2 - ( R * Id ) + ( L * Iq ) ]
  note: Iq = [ w / ( L * s ) ] * [ Vq1 - Vq2 - ( R * Iq ) - ( L * Id ) ]
  note: where w = 2*pi*Fnom (Hz)
  note: Vd1 - Vd2 = [ R * Id ] - [ L* w * Iq ] + [ L * d/dt (Id) ]
  note: o--------| R |---| L |-------o
  note: V1
  note: V2
  note: I --->
  note: ==========================================================================================
  note: Vq1 - Vq2 = [ R * Iq ] + [ L* w * Id ] + [ L * d/dt (Iq) ]
  note: where w = 2*pi*Fnom (Hz)
  Vdq1 : Inport
  Vdq2 : Inport  Port=2
  R_L : Inport  Port=3
  Demux3 : Demux  Outputs=2
      settings: DisplayOption=none
  Integrator : Integrator  InitialCondition="[I21_init_real   I21_init_imag]"
  Product : Product  SaturateOnIntegerOverflow=on  OutDataTypeStr=Inherit: Same as first input
  Product1 : Product  SaturateOnIntegerOverflow=on  OutDataTypeStr=Inherit: Same as first input
  Product2 : Product  Inputs=*/  SaturateOnIntegerOverflow=on  OutDataTypeStr=Inherit: Same as first input
  R_choke2 : Gain  Gain=[1 -1]  SaturateOnIntegerOverflow=on  OutDataTypeStr=Inherit: Same as input  ParamDataTypeStr=Inherit: Same as input
  R_choke3 : Gain  Gain=w  SaturateOnIntegerOverflow=on  OutDataTypeStr=Inherit: Same as input  ParamDataTypeStr=Inherit: Same as input
  Selector : Selector  InputPortWidth=2  IndexOptions=Index vector (dialog)  Indices=[2 1]  OutputSizes=1
  Sum : Sum  Inputs=+--+  SaturateOnIntegerOverflow=on
  idIq : Outport  VectorParamsAs1DForOutWhenUnconnected=off
  wires:
  Vdq1/1 -> Sum/1
  Vdq2/1 -> Sum/2
  Product/1 -> Sum/3
  R_choke2/1 -> Sum/4
  Product1/1 -> R_choke2/1
  Sum/1 -> R_choke3/1
  Integrator/1 -> idIq/1, Selector/1, Product/1
  Selector/1 -> Product1/1
  R_choke3/1 -> Product2/1
  Product2/1 -> Integrator/1
  R_L/1 -> Demux3/1
  Demux3/2 -> Product2/2, Product1/2
  Demux3/1 -> Product/2

== system LoadLevel1_VF/Three-Phase OLTC Regulating Transformer (Phasor Type)2/ Currents /dq0 model of 3-ph RL branch/Zero-sequence dq0 model of a 3-phase series R-L branch ==
  note: Using Laplace transform and per unit (pu) quantities :
  note: d-q axis model of a 3-phase series R-L branch
  note: Id = [ w / ( L * s ) ] * [ Vd1 - Vd2 - ( R * Id ) + ( L * Iq ) ]
  note: Iq = [ w / ( L * s ) ] * [ Vq1 - Vq2 - ( R * Iq ) - ( L * Id ) ]
  note: where w = 2*pi*Fnom (Hz)
  note: Vd1 - Vd2 = [ R * Id ] - [ L* w * Iq ] + [ L * d/dt (Id) ]
  note: o--------| R |---| L |-------o
  note: V1
  note: V2
  note: I --->
  note: ==========================================================================================
  note: Vq1 - Vq2 = [ R * Iq ] + [ L* w * Id ] + [ L * d/dt (Iq) ]
  note: where w = 2*pi*Fnom (Hz)
  Vdq1 : Inport
  Vdq2 : Inport  Port=2
  R_L : Inport  Port=3
  Demux3 : Demux  Outputs=2
      settings: DisplayOption=none
  Integrator : Integrator
  Product : Product  SaturateOnIntegerOverflow=on  OutDataTypeStr=Inherit: Same as first input
  Product1 : Product  SaturateOnIntegerOverflow=on  OutDataTypeStr=Inherit: Same as first input
  Product2 : Product  Inputs=*/  SaturateOnIntegerOverflow=on  OutDataTypeStr=Inherit: Same as first input
  R_choke2 : Gain  Gain=[1 -1]  SaturateOnIntegerOverflow=on  OutDataTypeStr=Inherit: Same as input  ParamDataTypeStr=Inherit: Same as input
  R_choke3 : Gain  Gain=w  SaturateOnIntegerOverflow=on  OutDataTypeStr=Inherit: Same as input  ParamDataTypeStr=Inherit: Same as input
  Selector : Selector  InputPortWidth=2  IndexOptions=Index vector (dialog)  Indices=[2 1]  OutputSizes=1
  Sum : Sum  Inputs=+--+  SaturateOnIntegerOverflow=on
  idIq : Outport  VectorParamsAs1DForOutWhenUnconnected=off
  wires:
  Vdq1/1 -> Sum/1
  Vdq2/1 -> Sum/2
  Product/1 -> Sum/3
  R_choke2/1 -> Sum/4
  Product1/1 -> R_choke2/1
  Sum/1 -> R_choke3/1
  Integrator/1 -> idIq/1, Selector/1, Product/1
  Selector/1 -> Product1/1
  R_choke3/1 -> Product2/1
  Product2/1 -> Integrator/1
  R_L/1 -> Demux3/1
  Demux3/2 -> Product2/2, Product1/2
  Demux3/1 -> Product/2

== system LoadLevel1_VF/Three-Phase OLTC Regulating Transformer (Phasor Type)2/Tap Changer Control/Edge Detector/NEGATIVE Edge ==
  IN : Inport
  IN previous : Inport  Port=2
  Enable : EnablePort  PropagateVarSize=During execution
  Relational Operator1 : RelationalOperator  Operator=>
  OUT : Outport  VectorParamsAs1DForOutWhenUnconnected=off
  wires:
  Relational Operator1/1 -> OUT/1
  IN previous/1 -> Relational Operator1/1
  IN/1 -> Relational Operator1/2

== system LoadLevel1_VF/Three-Phase OLTC Regulating Transformer (Phasor Type)2/Tap Changer Control/Edge Detector/POSITIVE Edge ==
  IN : Inport
  IN previous : Inport  Port=2
  Enable : EnablePort  PropagateVarSize=During execution
  Relational Operator1 : RelationalOperator  Operator=>
  OUT : Outport  VectorParamsAs1DForOutWhenUnconnected=off
  wires:
  Relational Operator1/1 -> OUT/1
  IN previous/1 -> Relational Operator1/2
  IN/1 -> Relational Operator1/1

== system LoadLevel1_VF/Three-Phase OLTC Regulating Transformer (Phasor Type)2/Voltage regulator/On//Off Delay/OFF Delay ==
  note: ic=-inf
  IN : Inport
  clock : Inport  Port=2
  DELAY : Inport  Port=3
  Enable : EnablePort  PropagateVarSize=During execution
  Edge Detector : Subsystem  DialogController=POWERSYS.PowerSysDialog  mask(Edge Detector){model=Falling, ic=ic}
      mask prompts: model "Edge:"; ic "Input at t = -eps:"
      mask help:
      | This block compares its present input to its previous input.
      |
      | If the input  is a logic signal (TRUE (1) or FALSE (0), the output is a one-step boolean signal TRUE  when  the specified edge (Rising, Falling or Either)  is detected.
      |
      | This block can also be used to detect the slope polarity of a continuous signal. For example, if the specified edge is  "Rising", the output is TRUE as long as the slope of the input signal is positive.
      |
      | The input value at time preceding t=0 is specified by the parameter "Input at t=-eps"
      mask init: same as LoadLevel1_VF/Three-Phase OLTC Regulating Transformer (Phasor Type)2/Tap Changer Control/Edge Detector
      mask Help: This block is part of a subset of blocks in the Extras library that does not have documentation associated with it, other than the block mask description.
      mask TypeOptions model: Rising | Falling | Either
      mask Display: plot(0,0,100,100, X1,Y1,X2,Y2,X3,Y3,X4,Y4);
  Logical Operator : Logic  Operator=NOT  Inputs=1
  Logical Operator1 : Logic  OutDataTypeStr=boolean
  Logical Operator2 : Logic  Operator=NOT  Inputs=1
  Relational Operator : RelationalOperator  OutDataTypeStr=boolean
  Sample & Hold : Subsystem  DialogController=POWERSYS.PowerSysDialog  mask(Sample & Hold){ic=-1e99}
      mask prompts: ic "Initial condition:"
      mask help: The output follows input 1 (In) as long as input 2 (S) is TRUE (1) . The output is held when input 2 becomes FALSE (0). The output initial value is specified by the parameter "Initial condition".
      mask init:
      | power_initmask();
      mask Help: This block is part of a subset of blocks in the Extras library that does not have documentation associated with it, other than the block mask description.
      mask Display: disp('S/H')
  Sum : Sum  InputSameDT=on  SaturateOnIntegerOverflow=on  OutDataTypeStr=Inherit: Same as first input
  OUT : Outport  VectorParamsAs1DForOutWhenUnconnected=off
  wires:
  Sample & Hold/1("   ") -> Sum/1
  Sum/1 -> Relational Operator/2
  DELAY/1 -> Sum/2
  Relational Operator/1 -> Logical Operator1/2
  Logical Operator1/1 -> Logical Operator2/1
  Logical Operator2/1 -> OUT/1
  IN/1 -> Logical Operator/1, Edge Detector/1(In)
  Logical Operator/1 -> Logical Operator1/1
  clock/1 -> Relational Operator/1, Sample & Hold/1(In)
  Edge Detector/1(Out) -> Sample & Hold/2(S)

== system LoadLevel1_VF/Three-Phase OLTC Regulating Transformer (Phasor Type)2/Voltage regulator/On//Off Delay/ON Delay ==
  note: ic=-inf
  IN : Inport
  clock : Inport  Port=2
  DELAY : Inport  Port=3
  Enable : EnablePort  PropagateVarSize=During execution
  Edge Detector : Subsystem  DialogController=POWERSYS.PowerSysDialog  mask(Edge Detector){model=Rising, ic=ic}
      mask prompts: model "Edge:"; ic "Input at t = -eps:"
      mask help:
      | This block compares its present input to its previous input.
      |
      | If the input  is a logic signal (TRUE (1) or FALSE (0), the output is a one-step boolean signal TRUE  when  the specified edge (Rising, Falling or Either)  is detected.
      |
      | This block can also be used to detect the slope polarity of a continuous signal. For example, if the specified edge is  "Rising", the output is TRUE as long as the slope of the input signal is positive.
      |
      | The input value at time preceding t=0 is specified by the parameter "Input at t=-eps"
      mask init: same as LoadLevel1_VF/Three-Phase OLTC Regulating Transformer (Phasor Type)2/Tap Changer Control/Edge Detector
      mask Help: This block is part of a subset of blocks in the Extras library that does not have documentation associated with it, other than the block mask description.
      mask TypeOptions model: Rising | Falling | Either
      mask Display: plot(0,0,100,100, X1,Y1,X2,Y2,X3,Y3,X4,Y4);
  Logical Operator2 : Logic
  Relational Operator : RelationalOperator  OutDataTypeStr=boolean
  Sample & Hold : Subsystem  DialogController=POWERSYS.PowerSysDialog  mask(Sample & Hold){ic=-1e99}
      mask prompts: ic "Initial condition:"
      mask help: The output follows input 1 (In) as long as input 2 (S) is TRUE (1) . The output is held when input 2 becomes FALSE (0). The output initial value is specified by the parameter "Initial condition".
      mask init:
      | power_initmask();
      mask Help: This block is part of a subset of blocks in the Extras library that does not have documentation associated with it, other than the block mask description.
      mask Display: disp('S/H')
  Sum : Sum  InputSameDT=on  SaturateOnIntegerOverflow=on  OutDataTypeStr=Inherit: Same as first input
  OUT : Outport  VectorParamsAs1DForOutWhenUnconnected=off
  wires:
  Sample & Hold/1("   ") -> Sum/1
  Edge Detector/1(Out) -> Sample & Hold/2(S)
  Relational Operator/1 -> Logical Operator2/1
  DELAY/1 -> Sum/2
  Sum/1 -> Relational Operator/2
  clock/1 -> Sample & Hold/1(In), Relational Operator/1
  IN/1 -> Edge Detector/1(In), Logical Operator2/2
  Logical Operator2/1 -> OUT/1

== system LoadLevel1_VF/Three-Phase OLTC Regulating Transformer (Phasor Type)2/Voltage regulator/On//Off Delay1/OFF Delay ==
  note: ic=-inf
  IN : Inport
  clock : Inport  Port=2
  DELAY : Inport  Port=3
  Enable : EnablePort  PropagateVarSize=During execution
  Edge Detector : Subsystem  DialogController=POWERSYS.PowerSysDialog  mask(Edge Detector){model=Falling, ic=ic}
      mask prompts: model "Edge:"; ic "Input at t = -eps:"
      mask help:
      | This block compares its present input to its previous input.
      |
      | If the input  is a logic signal (TRUE (1) or FALSE (0), the output is a one-step boolean signal TRUE  when  the specified edge (Rising, Falling or Either)  is detected.
      |
      | This block can also be used to detect the slope polarity of a continuous signal. For example, if the specified edge is  "Rising", the output is TRUE as long as the slope of the input signal is positive.
      |
      | The input value at time preceding t=0 is specified by the parameter "Input at t=-eps"
      mask init: same as LoadLevel1_VF/Three-Phase OLTC Regulating Transformer (Phasor Type)2/Tap Changer Control/Edge Detector
      mask Help: This block is part of a subset of blocks in the Extras library that does not have documentation associated with it, other than the block mask description.
      mask TypeOptions model: Rising | Falling | Either
      mask Display: plot(0,0,100,100, X1,Y1,X2,Y2,X3,Y3,X4,Y4);
  Logical Operator : Logic  Operator=NOT  Inputs=1
  Logical Operator1 : Logic  OutDataTypeStr=boolean
  Logical Operator2 : Logic  Operator=NOT  Inputs=1
  Relational Operator : RelationalOperator  OutDataTypeStr=boolean
  Sample & Hold : Subsystem  DialogController=POWERSYS.PowerSysDialog  mask(Sample & Hold){ic=-1e99}
      mask prompts: ic "Initial condition:"
      mask help: The output follows input 1 (In) as long as input 2 (S) is TRUE (1) . The output is held when input 2 becomes FALSE (0). The output initial value is specified by the parameter "Initial condition".
      mask init:
      | power_initmask();
      mask Help: This block is part of a subset of blocks in the Extras library that does not have documentation associated with it, other than the block mask description.
      mask Display: disp('S/H')
  Sum : Sum  InputSameDT=on  SaturateOnIntegerOverflow=on  OutDataTypeStr=Inherit: Same as first input
  OUT : Outport  VectorParamsAs1DForOutWhenUnconnected=off
  wires:
  Sample & Hold/1("   ") -> Sum/1
  Sum/1 -> Relational Operator/2
  DELAY/1 -> Sum/2
  Relational Operator/1 -> Logical Operator1/2
  Logical Operator1/1 -> Logical Operator2/1
  Logical Operator2/1 -> OUT/1
  IN/1 -> Logical Operator/1, Edge Detector/1(In)
  Logical Operator/1 -> Logical Operator1/1
  clock/1 -> Relational Operator/1, Sample & Hold/1(In)
  Edge Detector/1(Out) -> Sample & Hold/2(S)

== system LoadLevel1_VF/Three-Phase OLTC Regulating Transformer (Phasor Type)2/Voltage regulator/On//Off Delay1/ON Delay ==
  note: ic=-inf
  IN : Inport
  clock : Inport  Port=2
  DELAY : Inport  Port=3
  Enable : EnablePort  PropagateVarSize=During execution
  Edge Detector : Subsystem  DialogController=POWERSYS.PowerSysDialog  mask(Edge Detector){model=Rising, ic=ic}
      mask prompts: model "Edge:"; ic "Input at t = -eps:"
      mask help:
      | This block compares its present input to its previous input.
      |
      | If the input  is a logic signal (TRUE (1) or FALSE (0), the output is a one-step boolean signal TRUE  when  the specified edge (Rising, Falling or Either)  is detected.
      |
      | This block can also be used to detect the slope polarity of a continuous signal. For example, if the specified edge is  "Rising", the output is TRUE as long as the slope of the input signal is positive.
      |
      | The input value at time preceding t=0 is specified by the parameter "Input at t=-eps"
      mask init: same as LoadLevel1_VF/Three-Phase OLTC Regulating Transformer (Phasor Type)2/Tap Changer Control/Edge Detector
      mask Help: This block is part of a subset of blocks in the Extras library that does not have documentation associated with it, other than the block mask description.
      mask TypeOptions model: Rising | Falling | Either
      mask Display: plot(0,0,100,100, X1,Y1,X2,Y2,X3,Y3,X4,Y4);
  Logical Operator2 : Logic
  Relational Operator : RelationalOperator  OutDataTypeStr=boolean
  Sample & Hold : Subsystem  DialogController=POWERSYS.PowerSysDialog  mask(Sample & Hold){ic=-1e99}
      mask prompts: ic "Initial condition:"
      mask help: The output follows input 1 (In) as long as input 2 (S) is TRUE (1) . The output is held when input 2 becomes FALSE (0). The output initial value is specified by the parameter "Initial condition".
      mask init:
      | power_initmask();
      mask Help: This block is part of a subset of blocks in the Extras library that does not have documentation associated with it, other than the block mask description.
      mask Display: disp('S/H')
  Sum : Sum  InputSameDT=on  SaturateOnIntegerOverflow=on  OutDataTypeStr=Inherit: Same as first input
  OUT : Outport  VectorParamsAs1DForOutWhenUnconnected=off
  wires:
  Sample & Hold/1("   ") -> Sum/1
  Edge Detector/1(Out) -> Sample & Hold/2(S)
  Relational Operator/1 -> Logical Operator2/1
  DELAY/1 -> Sum/2
  Sum/1 -> Relational Operator/2
  clock/1 -> Sample & Hold/1(In), Relational Operator/1
  IN/1 -> Edge Detector/1(In), Logical Operator2/2
  Logical Operator2/1 -> OUT/1
